simulink model "taller6"  (R2025b)
settings: Solver=ode4  StartTime=0.0  StopTime=10.0  FixedStep=0.0001  RelTol=1e-3
settings Model: Creator=pedro  LastModifiedBy=pedro

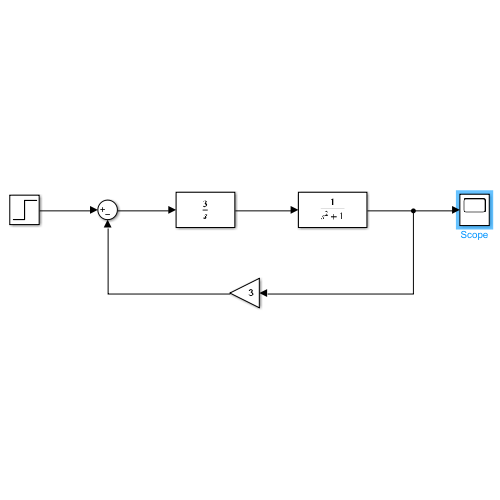
[thumbnail: Simulink's stored preview of the top-level diagram]
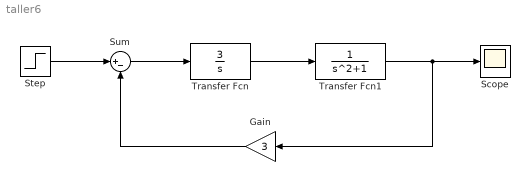
== system taller6 ==
  Gain : Gain  Gain=3
  Scope : Scope
      settings: ActiveDisplayYMinimum=-3192.3504952629464  ActiveDisplayYMaximum=1006.6964701767695
  Step : Step  Time=0  SampleTime=0
  Sum : Sum  Inputs=|+-
  Transfer Fcn : TransferFcn  Numerator=[3]  Denominator=[1 0]
  Transfer Fcn1 : TransferFcn  Denominator=[1 0 1]
  wires:
  Transfer Fcn/1 -> Transfer Fcn1/1
  Sum/1 -> Transfer Fcn/1
  Step/1 -> Sum/1
  Gain/1 -> Sum/2
  Transfer Fcn1/1 -> Gain/1, Scope/1
